simulink model "ACC_HW3"  (R2018b)
settings: Solver=ode2  StartTime=0.0  StopTime=endTime  FixedStep=Ts  RelTol=1e-3
undefined symbols (not defined in the file or in its folder): dSafe, Ts, v0_host, vref_host, x0_host
libraries: simulink x1
settings Model: Creator=jyotirmoy  LastModifiedBy=Administrator
settings SFSimCC: SimUseLocalCustomCode=off
settings RTWCC: RTWUseLocalCustomCode=off
settings CodeAppCC: StateflowObjectComments=on

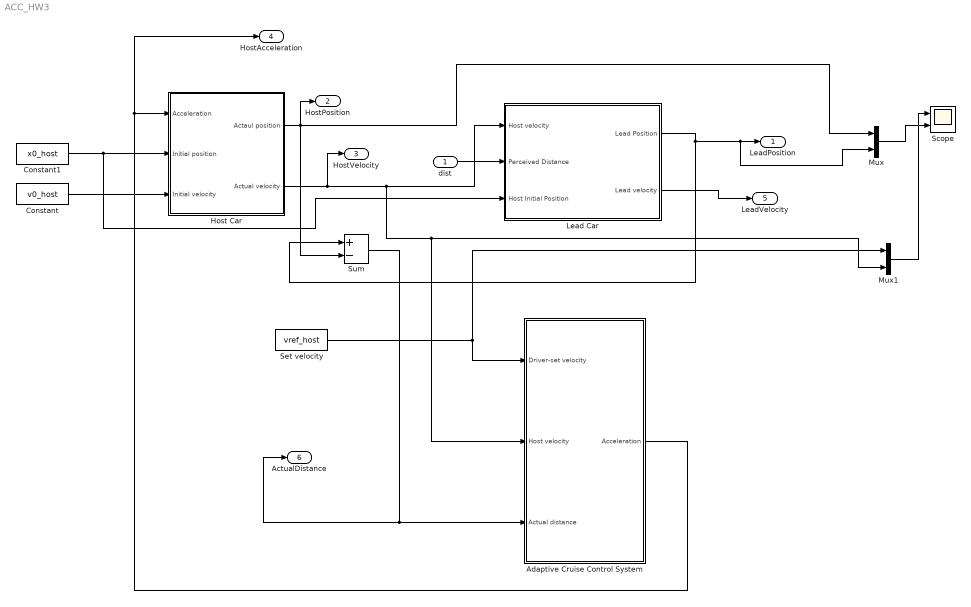
== system ACC_HW3 ==
  dist : Inport
  Adaptive Cruise Control System : Subsystem  VariantControl=MODE==4
  Constant : Constant  Value=v0_host
  Constant1 : Constant  Value=x0_host
  Host Car : Subsystem
  Lead Car : Subsystem
  Mux : Mux  Inputs=2
  Mux1 : Mux  Inputs=2
  Scope : Scope  NumInputPorts=2
  Set velocity : Constant  Value=vref_host  SampleTime=Ts
  Sum : Sum  Inputs=+-
  LeadPosition : Outport
  HostPosition : Outport  Port=2
  HostVelocity : Outport  Port=3
  HostAcceleration : Outport  Port=4
  LeadVelocity : Outport  Port=5
  ActualDistance : Outport  Port=6
  wires:
  Host Car/1(Actaul position) -> Mux/1, Sum/2, HostPosition/1
  Set velocity/1 -> Adaptive Cruise Control System/1(Driver-set velocity), Mux1/1
  Sum/1 -> ActualDistance/1, Adaptive Cruise Control System/3(Actual distance)
  Host Car/2(Actual velocity) -> Adaptive Cruise Control System/2(Host velocity), Mux1/2, Lead Car/1(Host velocity), HostVelocity/1
  Constant/1 -> Host Car/3(Initial velocity)
  Constant1/1 -> Lead Car/3(Host Initial Position), Host Car/2(Initial position)
  Lead Car/1(Lead Position) -> Mux/2, LeadPosition/1, Sum/1
  Mux/1 -> Scope/2
  Mux1/1 -> Scope/1
  Lead Car/2(Lead velocity) -> LeadVelocity/1
  dist/1 -> Lead Car/2(Perceived Distance)
  Adaptive Cruise Control System/1("Acceleration ") -> Host Car/1(Acceleration), HostAcceleration/1

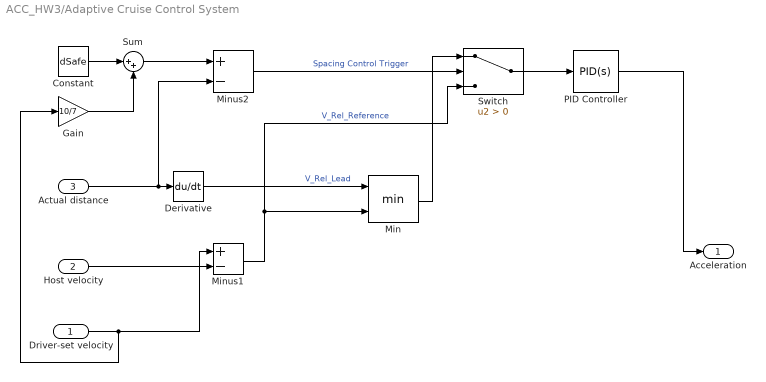
== system ACC_HW3/Adaptive Cruise Control System ==
  Driver-set velocity : Inport
  Host velocity : Inport  Port=2
  Actual distance : Inport  Port=3
  Constant : Constant  Value=dSafe
  Derivative : Derivative
  Gain : Gain  Gain=10/7
  Min : MinMax  Inputs=2
  Minus1 : Sum  Inputs=+-
  Minus2 : Sum  Inputs=+-
  PID Controller : simulink/Continuous/PID Controller  Controller=PID  Form=Parallel  TimeDomain=Continuous-time  SampleTime=-1  IntegratorMethod=Forward Euler  FilterMethod=Forward Euler  ControllerParametersSource=internal  P=0.7  I=0  D=0  UseFilter=on  N=100  TunerSelectOption=Transfer Function Based (PID Tuner App)  InitialConditionSource=internal  InitialConditionForIntegrator=0  InitialConditionForFilter=0  DifferentiatorICPrevScaledInput=0  ExternalReset=none  TrackingMode=off  Kt=1  LimitOutput=off  UpperSaturationLimit=inf  LowerSaturationLimit=-inf  LinearizeAsGain=on  AntiWindupMode=none  Kb=1  POutMin=[]  POutMax=[]  IOutMin=[]  IOutMax=[]  DOutMin=[]  DOutMax=[]  NOutMin=[]  NOutMax=[]  SumOutMin=[]  SumOutMax=[]  SaturationOutMin=[]  SaturationOutMax=[]  PParamMin=[]  PParamMax=[]  IParamMin=[]  IParamMax=[]  DParamMin=[]  DParamMax=[]  NParamMin=[]  NParamMax=[]  KbParamMin=[]  KbParamMax=[]  KtParamMin=[]  KtParamMax=[]  KbOutMin=[]  KbOutMax=[]  KtOutMin=[]  KtOutMax=[]  IntegratorOutMin=[]  IntegratorOutMax=[]  FilterOutMin=[]  FilterOutMax=[]  SumI1OutMin=[]  SumI1OutMax=[]  SumI2OutMin=[]  SumI2OutMax=[]  SumI3OutMin=[]  SumI3OutMax=[]  SumI4OutMin=[]  SumI4OutMax=[]  SumDOutMin=[]  SumDOutMax=[]  DifferentiatorOutMin=[]  DifferentiatorOutMax=[]  FilterDiffOutCoefMin=[]  FilterDiffOutCoefMax=[]  ReciprocalOutMin=[]  ReciprocalOutMax=[]  SumDenOutMin=[]  SumDenOutMax=[]  SumNumOutMin=[]  SumNumOutMax=[]  DivideOutMin=[]  DivideOutMax=[]  IntegratorContinuousStateAttributes=''  IntegratorStateMustResolveToSignalObject=off  IntegratorRTWStateStorageClass=Auto  FilterContinuousStateAttributes=''  FilterStateMustResolveToSignalObject=off  FilterRTWStateStorageClass=Auto  ParallelPVariant=InternalParameters  IdealPVariant=Disabled  IVariant=InternalParameters  DVariant=InternalParameters  IntegratorVariant=Continuous  SatVariant=Disabled  AWVariant=Passthrough  PCopyVariant=Disabled  TRVariant=Disabled  FdbkBlocksVariant=Forward  IdealPFdbkVariant=Disabled  SatFdbkVariant=Disabled  DerivativeFilterVariant=ContFilter  NVariant=InternalParameters  NCopyVariant=Disabled  FilterICVariant=InternalICsFilter  IntegratorICVariant=InternalICs  ExternalResetVariant=Disabled  TRSumVariant=Passthrough  SumFdbkVariant=Disabled  SumVariant=Sum_PID
  Sum : Sum  Inputs=|++
  Switch : Switch  Criteria=u2 > Threshold
  "Acceleration " : Outport
  wires:
  Driver-set velocity/1 -> Gain/1, Minus1/1
  Host velocity/1 -> Minus1/2
  Switch/1 -> PID Controller/1
  Derivative/1 -> Min/1  "V_Rel_Lead"
  PID Controller/1 -> "Acceleration "/1
  Constant/1 -> Sum/1
  Actual distance/1 -> Minus2/2, Derivative/1
  Minus1/1 -> Switch/3, Min/2  "V_Rel_Reference"
  Sum/1 -> Minus2/1
  Gain/1 -> Sum/2
  Min/1 -> Switch/1
  Minus2/1 -> Switch/2  "Spacing Control Trigger"

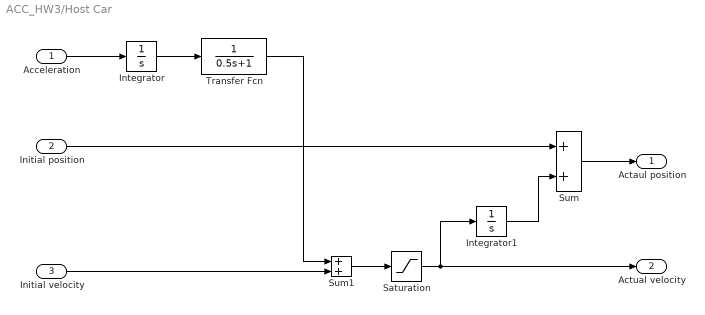
== system ACC_HW3/Host Car ==
  Acceleration : Inport
  Initial position : Inport  Port=2
  Initial velocity : Inport  Port=3
  Integrator : Integrator
  Integrator1 : Integrator
  Saturation : Saturate  UpperLimit=vref_host  LowerLimit=0
  Sum : Sum
  Sum1 : Sum
  Transfer Fcn : TransferFcn  Denominator=[0.5 1]
  Actaul position : Outport
  Actual velocity : Outport  Port=2
  wires:
  Initial velocity/1 -> Sum1/2
  Sum/1 -> Actaul position/1
  Transfer Fcn/1 -> Sum1/1
  Integrator/1 -> Transfer Fcn/1
  Acceleration/1 -> Integrator/1
  Initial position/1 -> Sum/1
  Integrator1/1 -> Sum/2
  Sum1/1 -> Saturation/1
  Saturation/1 -> Actual velocity/1, Integrator1/1

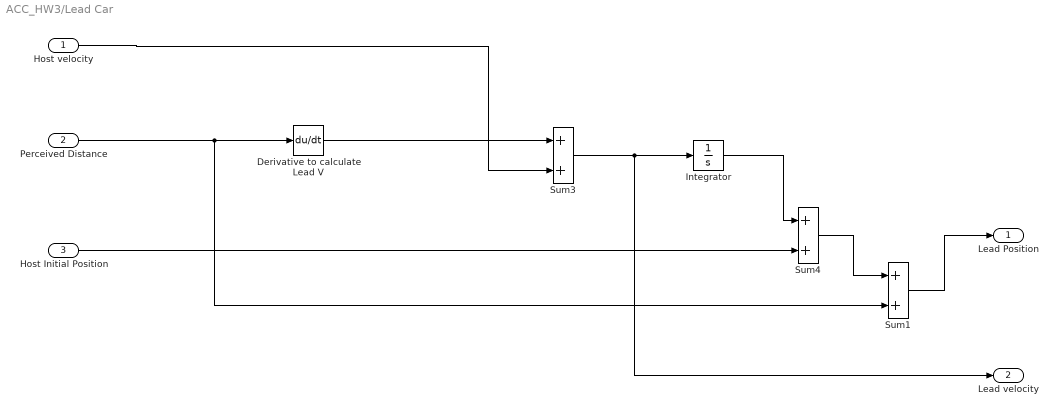
== system ACC_HW3/Lead Car ==
  Host velocity : Inport
  Perceived Distance : Inport  Port=2
  Host Initial Position : Inport  Port=3
  Derivative to calculate Lead V : Derivative
  Integrator : Integrator
  Sum1 : Sum
  Sum3 : Sum
  Sum4 : Sum
  Lead Position : Outport
  Lead velocity : Outport  Port=2
  wires:
  Sum4/1 -> Sum1/1
  Sum3/1 -> Lead velocity/1, Integrator/1
  Host velocity/1 -> Sum3/2
  Derivative to calculate Lead V/1 -> Sum3/1
  Host Initial Position/1 -> Sum4/2
  Integrator/1 -> Sum4/1
  Perceived Distance/1 -> Sum1/2, Derivative to calculate Lead V/1
  Sum1/1 -> Lead Position/1
